simulink model "gm_CodeGeneration"  (R2017a)
settings: Solver=VariableStepAuto  StartTime=0.0  StopTime=10.0  RelTol=1e-3
settings Model: Creator=Arthur  LastModifiedBy=Arthur
settings OptimizationCC: BlockReduction=off  ConditionallyExecuteInputs=off
settings DebuggingCC: InheritedTsInSrcMsg=none

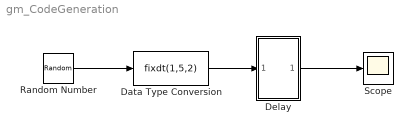
== system gm_CodeGeneration ==
  Data Type Conversion : DataTypeConversion  OutDataTypeStr=fixdt(1,5,2)
  Delay : Subsystem
  Random Number : RandomNumber  SampleTime=0.1
  Scope : Scope
  wires:
  Delay/1(Out1) -> Scope/1
  Data Type Conversion/1 -> Delay/1(In1)
  Random Number/1 -> Data Type Conversion/1

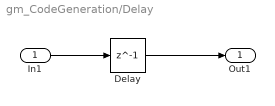
== system gm_CodeGeneration/Delay ==
  In1 : Inport
  Delay : Delay  DelayLength=1
  Out1 : Outport
  wires:
  In1/1 -> Delay/1
  Delay/1 -> Out1/1
